simulink model "MIT_bosung"  (Simulink 7.3)
settings: Solver=ode5  StartTime=0.0  StopTime=100  FixedStep=0.0001  RelTol=1e-3
StopFcn:
  | subplot(211);
  | plot(Data.time,Data.signals(1).values(:,1),'r',Data.time,Data.signals(1).values(:,2),'b')
  | subplot(212);
  | plot(Data.time,Data.signals(2).values(:,1),'b')
values from neighbouring files (symbols this model uses):
  T = 0.001    [ARMA_vs_Correlogram.m]    (also in AR_model_LS_AIC.m; AR_model_LS_BIC.m; AR_model_LS_PFE.m; AR_model_YW.m)
undefined symbols (not defined in the file or in its folder): k
libraries: simulink x1
settings Model: Creator=Minh-Map-Vu  LastModifiedBy=nthuy
settings DataIOCC: SignalLoggingName=sigsOut
settings DebuggingCC: SaveWithParameterizedLinksMsg=none  SignalResolutionControl=TryResolveAllWithWarning  SolverPrmCheckMsg=none  MultiTaskDSMMsg=warning  MultiTaskCondExecSysMsg=none  StrictBusMsg=None
settings HardwareCC: TargetEndianess=LittleEndian  TargetHWDeviceType=MATLAB Host  ProdEqTarget=off
settings RTWCC: IncludeERTFirstTime=on

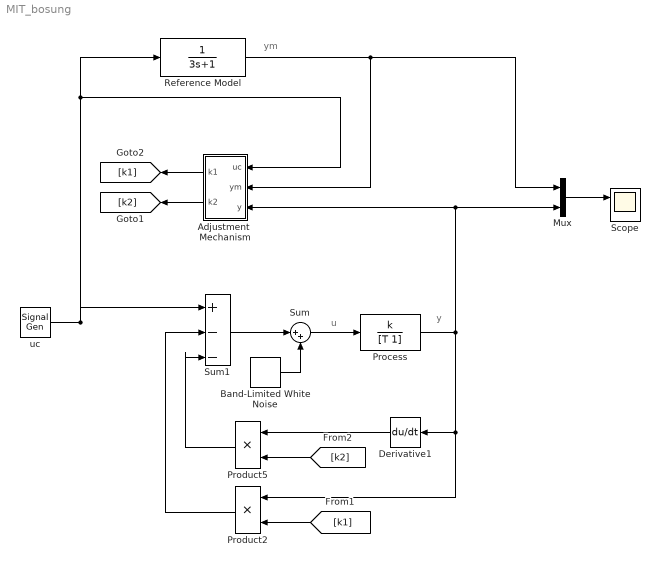
== system MIT_bosung ==
  note: ym
  note: u
  note: y
  Adjustment  Mechanism : Subsystem
  Band-Limited White Noise : simulink/Sources/Band-Limited White Noise  SystemSampleTime=-1  Cov=[0.01]  Ts=0.0001  seed=[23341]
  Derivative1 : Derivative
  Mux : Mux  Inputs=2
  Process : TransferFcn  Numerator=k  Denominator=[T 1]
  Product2 : Product  SaturateOnIntegerOverflow=on  OutDataTypeStr=Inherit: Same as first input
  Product5 : Product  SaturateOnIntegerOverflow=on  OutDataTypeStr=Inherit: Same as first input
  Reference Model : TransferFcn  Denominator=[3 1]
  Scope : Scope  NumInputPorts=2
      settings: TimeRange=100  YMin=-1.2~-5  YMax=1.2~5  SaveName=Data
  Sum : Sum  Inputs=|++  OutDataType=fixdt(1, 16)  OutScaling=2^0
  Sum1 : Sum  Inputs=|+--  SaturateOnIntegerOverflow=on
  uc : SignalGenerator  WaveForm=square  Frequency=1/20
  wires:
  uc/1 -> Sum1/1, Reference Model/1, Adjustment  Mechanism/1(uc)
  Reference Model/1 -> Mux/1, Adjustment  Mechanism/2(ym)
  Process/1 -> Derivative1/1, Product2/1, Mux/2, Adjustment  Mechanism/3(y)
  [k1] -> Product2/2
  Product2/1 -> Sum1/2
  [k2] -> Product5/2
  Derivative1/1 -> Product5/1
  Product5/1 -> Sum1/3
  Adjustment  Mechanism/1(k1) -> [k1]
  Adjustment  Mechanism/2(k2) -> [k2]
  Mux/1 -> Scope/1
  Sum1/1 -> Sum/1
  Sum/1 -> Process/1
  Band-Limited White Noise/1 -> Sum/2

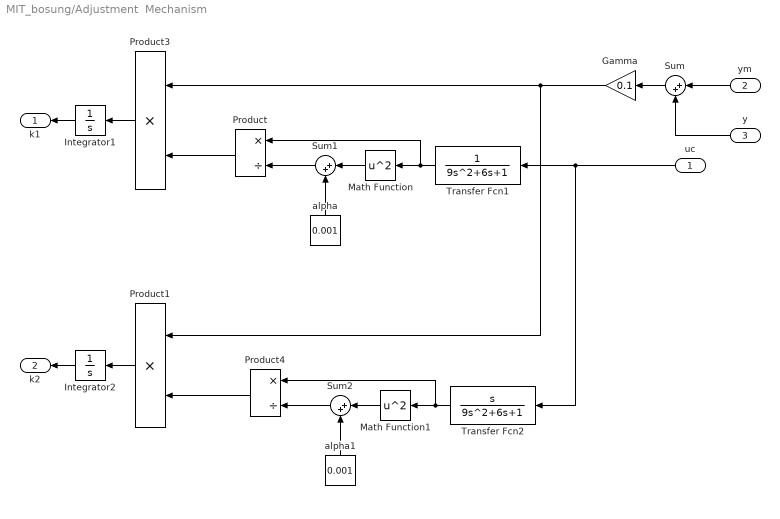
== system MIT_bosung/Adjustment  Mechanism ==
  uc : Inport  OutDataType=fixdt(1, 16)  OutScaling=2^0
  ym : Inport  Port=2  OutDataType=fixdt(1, 16)  OutScaling=2^0
  y : Inport  Port=3  OutDataType=fixdt(1, 16)  OutScaling=2^0
  Gamma : Gain  Gain=0.1  ParameterDataType=fixdt(1, 16)  ParameterScaling=2^0  OutDataType=fixdt(1, 16)  OutScaling=2^0
  Integrator1 : Integrator
  Integrator2 : Integrator
  Math Function : Math  Operator=square  OutDataType=fixdt(1, 16)  OutScaling=2^0  SaturateOnIntegerOverflow=on
  Math Function1 : Math  Operator=square  OutDataType=fixdt(1, 16)  OutScaling=2^0  SaturateOnIntegerOverflow=on
  Product : Product  Inputs=*/  OutDataType=fixdt(1, 16)  OutScaling=2^0  RndMeth=Zero
  Product1 : Product  SaturateOnIntegerOverflow=on  OutDataTypeStr=Inherit: Same as first input
  Product3 : Product  SaturateOnIntegerOverflow=on  OutDataTypeStr=Inherit: Same as first input
  Product4 : Product  Inputs=*/  OutDataType=fixdt(1, 16)  OutScaling=2^0  RndMeth=Zero
  Sum : Sum  Inputs=|++  OutDataType=fixdt(1, 16)  OutScaling=2^0
  Sum1 : Sum  Inputs=|++  OutDataType=fixdt(1, 16)  OutScaling=2^0
  Sum2 : Sum  Inputs=|++  OutDataType=fixdt(1, 16)  OutScaling=2^0
  Transfer Fcn1 : TransferFcn  Denominator=[9 6 1]
  Transfer Fcn2 : TransferFcn  Numerator=[1 0]  Denominator=[9 6 1]
  alpha : Constant  Value=0.001  OutDataType=fixdt(1, 16)  OutScaling=2^0
  alpha1 : Constant  Value=0.001  OutDataType=fixdt(1, 16)  OutScaling=2^0
  k1 : Outport
  k2 : Outport  Port=2
  wires:
  Product3/1 -> Integrator1/1
  Product1/1 -> Integrator2/1
  Integrator1/1 -> k1/1
  Integrator2/1 -> k2/1
  ym/1 -> Sum/1
  y/1 -> Sum/2
  alpha/1 -> Sum1/2
  Sum1/1 -> Product/2
  Math Function/1 -> Sum1/1
  Transfer Fcn1/1 -> Math Function/1, Product/1
  Product/1 -> Product3/2
  uc/1 -> Transfer Fcn1/1, Transfer Fcn2/1
  alpha1/1 -> Sum2/2
  Sum2/1 -> Product4/2
  Math Function1/1 -> Sum2/1
  Transfer Fcn2/1 -> Math Function1/1, Product4/1
  Product4/1 -> Product1/2
  Sum/1 -> Gamma/1
  Gamma/1 -> Product3/1, Product1/1
